simulink model "base_simulink"  (R2022a)
settings: Solver=FixedStepAuto  StartTime=0.0  StopTime=20  FixedStep=0.00005  MaxStep=1e-4  RelTol=1e-5
model workspace (MAT data in the model file):
  SL_ROS_VariableLengthArrays_MaxSizes : object (value not decoded)
undefined symbols (not defined in the file): position, position_SL_Info, sigbuilder_block, twist, X, Y, Z
libraries: sm_lib x128, nesl_utility x42, slpidlib x16, ros2lib x12, dspstat3 x2, dspsigops x1
(part 6 of 6)

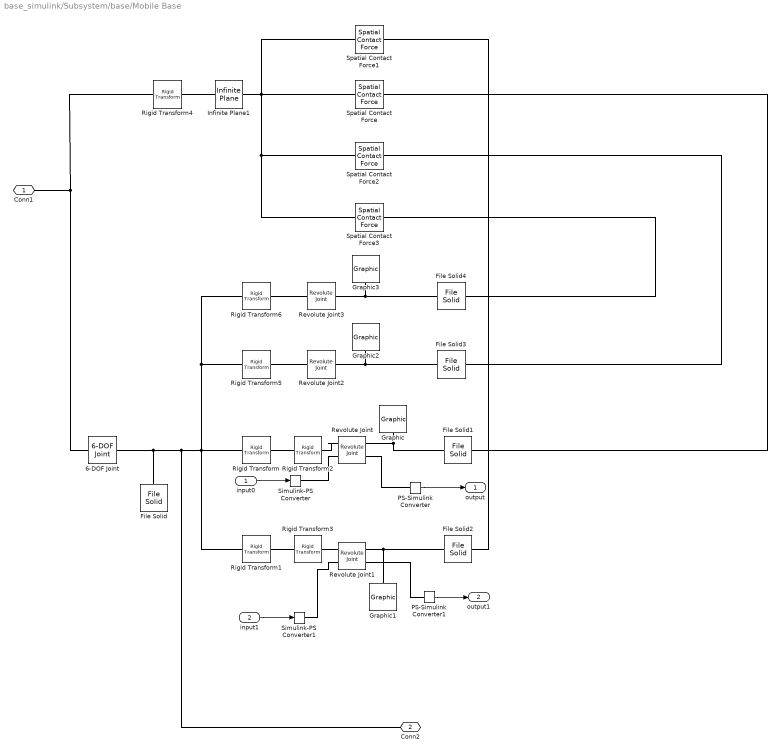
== system base_simulink/Subsystem/base/Mobile Base ==
  input0 : Inport
  input1 : Inport  Port=2
  6-DOF Joint : sm_lib/Joints/6-DOF Joint  JointMode=Normal  SenseConstraintForce=off  SenseConstraintForceX=off  SenseConstraintForceY=off  SenseConstraintForceZ=off  SenseConstraintTorque=off  SenseConstraintTorqueX=off  SenseConstraintTorqueY=off  SenseConstraintTorqueZ=off  SenseTotalForce=off  SenseTotalForceX=off  SenseTotalForceY=off  SenseTotalForceZ=off  SenseTotalTorque=off  SenseTotalTorqueX=off  SenseTotalTorqueY=off  SenseTotalTorqueZ=off  CompositeWrenchDir=FollowerOnBase  CompositeWrenchFrame=BaseFrame  PxEquilibriumPosition=0  PxEquilibriumPositionUnits=m  PxSpringStiffness=0  PxSpringStiffnessUnits=N/m  PxDampingCoefficient=0  PxDampingCoefficientUnits=N/(m/s)  PxTorqueActuationMode=NoTorque  PxMotionActuationMode=ComputedMotion  PxSensePosition=off  PxSenseVelocity=off  PxSenseAcceleration=off  PxSenseTorqueForce=off  PxSenseLowerLimitTorqueForce=off  PxSenseUpperLimitTorqueForce=off  PxLowerLimitSpecify=off  PxLowerLimitBound=-1  PxLowerLimitBoundUnits=m  PxLowerLimitStiffness=1e6  PxLowerLimitStiffnessUnits=N/m  PxLowerLimitDamping=1e3  PxLowerLimitDampingUnits=N/(m/s)  PxLowerLimitTransitionRegionWidth=1e-4  PxLowerLimitTransitionRegionWidthUnits=m  PxUpperLimitSpecify=off  PxUpperLimitBound=1  PxUpperLimitBoundUnits=m  PxUpperLimitStiffness=1e6  PxUpperLimitStiffnessUnits=N/m  PxUpperLimitDamping=1e3  PxUpperLimitDampingUnits=N/(m/s)  PxUpperLimitTransitionRegionWidth=1e-4  PxUpperLimitTransitionRegionWidthUnits=m  PxPositionTargetSpecify=off  PxPositionTargetPriority=High  PxPositionTargetValue=0  PxPositionTargetValueUnits=m  PxVelocityTargetSpecify=off  PxVelocityTargetPriority=High  PxVelocityTargetValue=0  PxVelocityTargetValueUnits=m/s  PyEquilibriumPosition=0  PyEquilibriumPositionUnits=m  PySpringStiffness=0  PySpringStiffnessUnits=N/m  PyDampingCoefficient=0  PyDampingCoefficientUnits=N/(m/s)  PyTorqueActuationMode=NoTorque  PyMotionActuationMode=ComputedMotion  PySensePosition=off  PySenseVelocity=off  PySenseAcceleration=off  PySenseTorqueForce=off  PySenseLowerLimitTorqueForce=off  PySenseUpperLimitTorqueForce=off  PyLowerLimitSpecify=off  PyLowerLimitBound=-1  PyLowerLimitBoundUnits=m  PyLowerLimitStiffness=1e6  PyLowerLimitStiffnessUnits=N/m  PyLowerLimitDamping=1e3  PyLowerLimitDampingUnits=N/(m/s)  PyLowerLimitTransitionRegionWidth=1e-4  PyLowerLimitTransitionRegionWidthUnits=m  PyUpperLimitSpecify=off  PyUpperLimitBound=1  PyUpperLimitBoundUnits=m  PyUpperLimitStiffness=1e6  PyUpperLimitStiffnessUnits=N/m  PyUpperLimitDamping=1e3  PyUpperLimitDampingUnits=N/(m/s)  PyUpperLimitTransitionRegionWidth=1e-4  PyUpperLimitTransitionRegionWidthUnits=m  PyPositionTargetSpecify=off  PyPositionTargetPriority=High  PyPositionTargetValue=0  PyPositionTargetValueUnits=m  PyVelocityTargetSpecify=off  PyVelocityTargetPriority=High  PyVelocityTargetValue=0  PyVelocityTargetValueUnits=m/s  PzEquilibriumPosition=0  PzEquilibriumPositionUnits=m  PzSpringStiffness=0  PzSpringStiffnessUnits=N/m  PzDampingCoefficient=0  PzDampingCoefficientUnits=N/(m/s)  PzTorqueActuationMode=NoTorque  PzMotionActuationMode=ComputedMotion  PzSensePosition=off  PzSenseVelocity=off  PzSenseAcceleration=off  PzSenseTorqueForce=off  PzSenseLowerLimitTorqueForce=off  PzSenseUpperLimitTorqueForce=off  PzLowerLimitSpecify=off  PzLowerLimitBound=-1  PzLowerLimitBoundUnits=m  PzLowerLimitStiffness=1e6  PzLowerLimitStiffnessUnits=N/m  PzLowerLimitDamping=1e3  PzLowerLimitDampingUnits=N/(m/s)  PzLowerLimitTransitionRegionWidth=1e-4  PzLowerLimitTransitionRegionWidthUnits=m  PzUpperLimitSpecify=off  PzUpperLimitBound=1  PzUpperLimitBoundUnits=m  PzUpperLimitStiffness=1e6  PzUpperLimitStiffnessUnits=N/m  PzUpperLimitDamping=1e3  PzUpperLimitDampingUnits=N/(m/s)  PzUpperLimitTransitionRegionWidth=1e-4  PzUpperLimitTransitionRegionWidthUnits=m  PzPositionTargetSpecify=off  PzPositionTargetPriority=High  PzPositionTargetValue=0  PzPositionTargetValueUnits=m  PzVelocityTargetSpecify=off  PzVelocityTargetPriority=High  PzVelocityTargetValue=0  PzVelocityTargetValueUnits=m/s  SphDefPosRotationMethod=None  SphDefPosRotationAngleUnits=deg  SphDefPosRotationStandardAxis=+Z  SphDefPosRotationAngle=0.0  SphDefPosRotationArbitraryAxis=[0 0 1]  SphDefPosFollAlignAxisA=+X  SphDefPosBaseAlignAxisA=+Y  SphDefPosFollAlignAxisB=+Y  SphDefPosBaseAlignAxisB=+Z  SphDefPosRotationSequenceAxes=FollowerAxes  SphDefPosRotationSequence=XYX  SphDefPosRotationSequenceAngles=[0 0 0]  SphDefPosRotationSequenceAnglesUnits=deg  SphDefPosRotationMatrix=[1 0 0; 0 1 0; 0 0 1]  SphEqPosRotationMethod=None  SphEqPosRotationAngleUnits=deg  SphEqPosRotationStandardAxis=+Z  SphEqPosRotationAngle=0.0  SphEqPosRotationArbitraryAxis=[0 0 1]  SphEqPosFollAlignAxisA=+X  SphEqPosBaseAlignAxisA=+Y  SphEqPosFollAlignAxisB=+Y  SphEqPosBaseAlignAxisB=+Z  SphEqPosRotationSequenceAxes=FollowerAxes  SphEqPosRotationSequence=XYX  SphEqPosRotationSequenceAngles=[0 0 0]  SphEqPosRotationSequenceAnglesUnits=deg  SphEqPosRotationMatrix=[1 0 0; 0 1 0; 0 0 1]  SphSpringStiffness=0  SphSpringStiffnessUnits=N*m/deg  SphDampingCoefficient=0  SphDampingCoefficientUnits=N*m/(deg/s)  SphActuateTorqueX=off  SphActuateTorqueY=off  SphActuateTorqueZ=off  SphActuateTorque=off  SphTorqueActuationMode=NoTorque  SphMotionActuationMode=ComputedMotion  SphActuationFrame=BaseFrame  SphSensePosition=off  SphSenseVelocityX=off  SphSenseVelocityY=off  SphSenseVelocityZ=off  SphSenseVelocity=off  SphSenseAccelerationX=off  SphSenseAccelerationY=off  SphSenseAccelerationZ=off  SphSenseAcceleration=off  SphSenseTorqueX=off  SphSenseTorqueY=off  SphSenseTorqueZ=off  SphSenseTorqueForce=off  SphSenseLowerLimitTorqueMag=off  SphSenseUpperLimitTorqueMag=off  SphSensingFrame=BaseFrame  SphLowerLimitSpecify=off  SphLowerLimitBound=15  SphLowerLimitBoundUnits=deg  SphLowerLimitStiffness=1e4  SphLowerLimitStiffnessUnits=N*m/deg  SphLowerLimitDamping=10  SphLowerLimitDampingUnits=N*m/(deg/s)  SphLowerLimitTransitionRegionWidth=0.1  SphLowerLimitTransitionRegionWidthUnits=deg  SphUpperLimitSpecify=off  SphUpperLimitBound=45  SphUpperLimitBoundUnits=deg  SphUpperLimitStiffness=1e4  SphUpperLimitStiffnessUnits=N*m/deg  SphUpperLimitDamping=10  SphUpperLimitDampingUnits=N*m/(deg/s)  SphUpperLimitTransitionRegionWidth=0.1  SphUpperLimitTransitionRegionWidthUnits=deg  SphPositionTargetRotationMethod=None  SphPositionTargetRotationAngleUnits=deg  SphPositionTargetRotationStandardAxis=+Z  SphPositionTargetRotationAngle=0.0  SphPositionTargetRotationArbitraryAxis=[0 0 1]  SphPositionTargetFollAlignAxisA=+X  SphPositionTargetBaseAlignAxisA=+Y  SphPositionTargetFollAlignAxisB=+Y  SphPositionTargetBaseAlignAxisB=+Z  SphPositionTargetRotationSequenceAxes=FollowerAxes  SphPositionTargetRotationSequence=XYX  SphPositionTargetRotationSequenceAngles=[0 0 0]  SphPositionTargetRotationSequenceAnglesUnits=deg  SphPositionTargetRotationMatrix=[1 0 0; 0 1 0; 0 0 1]  SphPositionTargetSpecify=off  SphPositionTargetPriority=High  SphVelocityTargetValue=[0 0 0]  SphVelocityTargetValueUnits=deg/s  SphVelocityTargetSpecify=off  SphVelocityTargetPriority=High  SphVelocityTargetInFollowerFrame=on
  File Solid : sm_lib/Body Elements/File Solid  ExtGeomFileName=C:\Users\matas\Desktop\FIBO4\FRA502MBSE\BASE_simulink\BASE_simulink\chassis.step  UnitType=FromFile  ExtGeomFileUnits=m  StepReaderType=HEX  ExportConvexHullGeometry=off  InertiaType=Custom  Mass=45.683  MassUnits=kg  CenterOfMass=[-117.99 2.46 415.85]  CenterOfMassUnits=mm  MomentsOfInertia=[16.23572765580 17.36819929236 2.01273191058]  MomentsOfInertiaUnits=kg*m^2  ProductsOfInertia=[0.10365361699 1.80624053893 0.02552226667]  ProductsOfInertiaUnits=kg*m^2  BasedOnType=DensityFromFile  Density=1000  DensityUnits=kg/m^3  DoExposeReferenceFrame=on  SerializedFrames=<Frames/>  GraphicType=FromGeometry  MarkerShape=Sphere  MarkerSize=10  GraphicVisPropType=SimpleVisualProperties  GraphicDiffuseColor=[0.5 0.5 0.5]  GraphicSpecularColor=[0.5 0.5 0.5 1.0]  GraphicAmbientColor=[0.15 0.15 0.15 1.0]  GraphicEmissiveColor=[0.0 0.0 0.0 1.0]  GraphicShininess=75  GraphicOpacity=1.0
  File Solid1 : sm_lib/Body Elements/File Solid  ExtGeomFileName=C:\Users\matas\Desktop\FIBO4\FRA502MBSE\BASE_simulink\BASE_simulink\wheel.step  UnitType=FromFile  ExtGeomFileUnits=m  StepReaderType=HEX  ExportConvexHullGeometry=on  InertiaType=CalculateFromGeometry  Mass=0.5  MassUnits=kg  CenterOfMass=[0 0 0]  CenterOfMassUnits=m  MomentsOfInertia=[1 1 1]  MomentsOfInertiaUnits=kg*m^2  ProductsOfInertia=[0 0 0]  ProductsOfInertiaUnits=kg*m^2  BasedOnType=Mass  Density=1000  DensityUnits=kg/m^3  DoExposeReferenceFrame=on  SerializedFrames=<Frames/>  GraphicType=FromGeometry  MarkerShape=Sphere  MarkerSize=10  GraphicVisPropType=SimpleVisualProperties  GraphicDiffuseColor=[0.5 0.5 0.5]  GraphicSpecularColor=[0.5 0.5 0.5 1.0]  GraphicAmbientColor=[0.15 0.15 0.15 1.0]  GraphicEmissiveColor=[0.0 0.0 0.0 1.0]  GraphicShininess=75  GraphicOpacity=1.0
  File Solid2 : sm_lib/Body Elements/File Solid  ExtGeomFileName=C:\Users\matas\Desktop\FIBO4\FRA502MBSE\BASE_simulink\BASE_simulink\wheel.step  UnitType=FromFile  ExtGeomFileUnits=m  StepReaderType=HEX  ExportConvexHullGeometry=on  InertiaType=CalculateFromGeometry  Mass=0.5  MassUnits=kg  CenterOfMass=[0 0 0]  CenterOfMassUnits=m  MomentsOfInertia=[1 1 1]  MomentsOfInertiaUnits=kg*m^2  ProductsOfInertia=[0 0 0]  ProductsOfInertiaUnits=kg*m^2  BasedOnType=Mass  Density=1000  DensityUnits=kg/m^3  DoExposeReferenceFrame=on  SerializedFrames=<Frames/>  GraphicType=FromGeometry  MarkerShape=Sphere  MarkerSize=10  GraphicVisPropType=SimpleVisualProperties  GraphicDiffuseColor=[0.5 0.5 0.5]  GraphicSpecularColor=[0.5 0.5 0.5 1.0]  GraphicAmbientColor=[0.15 0.15 0.15 1.0]  GraphicEmissiveColor=[0.0 0.0 0.0 1.0]  GraphicShininess=75  GraphicOpacity=1.0
  File Solid3 : sm_lib/Body Elements/File Solid  ExtGeomFileName=C:\Users\matas\Desktop\FIBO4\FRA502MBSE\BASE_simulink\BASE_simulink\caster wheel.step  UnitType=FromFile  ExtGeomFileUnits=m  StepReaderType=HEX  ExportConvexHullGeometry=on  InertiaType=CalculateFromGeometry  Mass=1  MassUnits=kg  CenterOfMass=[0 0 0]  CenterOfMassUnits=m  MomentsOfInertia=[1 1 1]  MomentsOfInertiaUnits=kg*m^2  ProductsOfInertia=[0 0 0]  ProductsOfInertiaUnits=kg*m^2  BasedOnType=Mass  Density=1000  DensityUnits=kg/m^3  DoExposeReferenceFrame=on  SerializedFrames=<Frames/>  GraphicType=FromGeometry  MarkerShape=Sphere  MarkerSize=10  GraphicVisPropType=SimpleVisualProperties  GraphicDiffuseColor=[0.5 0.5 0.5]  GraphicSpecularColor=[0.5 0.5 0.5 1.0]  GraphicAmbientColor=[0.15 0.15 0.15 1.0]  GraphicEmissiveColor=[0.0 0.0 0.0 1.0]  GraphicShininess=75  GraphicOpacity=1.0
  File Solid4 : sm_lib/Body Elements/File Solid  ExtGeomFileName=C:\Users\matas\Desktop\FIBO4\FRA502MBSE\BASE_simulink\BASE_simulink\caster wheel.step  UnitType=FromFile  ExtGeomFileUnits=m  StepReaderType=HEX  ExportConvexHullGeometry=on  InertiaType=CalculateFromGeometry  Mass=1  MassUnits=kg  CenterOfMass=[0 0 0]  CenterOfMassUnits=m  MomentsOfInertia=[1 1 1]  MomentsOfInertiaUnits=kg*m^2  ProductsOfInertia=[0 0 0]  ProductsOfInertiaUnits=kg*m^2  BasedOnType=Mass  Density=1000  DensityUnits=kg/m^3  DoExposeReferenceFrame=on  SerializedFrames=<Frames/>  GraphicType=FromGeometry  MarkerShape=Sphere  MarkerSize=10  GraphicVisPropType=SimpleVisualProperties  GraphicDiffuseColor=[0.5 0.5 0.5]  GraphicSpecularColor=[0.5 0.5 0.5 1.0]  GraphicAmbientColor=[0.15 0.15 0.15 1.0]  GraphicEmissiveColor=[0.0 0.0 0.0 1.0]  GraphicShininess=75  GraphicOpacity=1.0
  Graphic : sm_lib/Body Elements/Graphic  GraphicType=Marker  MarkerShape=Frame  MarkerSize=20  GraphicVisPropType=SimpleVisualProperties  GraphicDiffuseColor=[0 1 0]  GraphicSpecularColor=[0.5 0.5 0.5 1.0]  GraphicAmbientColor=[0.15 0.15 0.15 1.0]  GraphicEmissiveColor=[0.0 0.0 0.0 1.0]  GraphicShininess=75  GraphicOpacity=1.0
  Graphic1 : sm_lib/Body Elements/Graphic  GraphicType=Marker  MarkerShape=Frame  MarkerSize=20  GraphicVisPropType=SimpleVisualProperties  GraphicDiffuseColor=[1 0 0]  GraphicSpecularColor=[0.5 0.5 0.5 1.0]  GraphicAmbientColor=[0.15 0.15 0.15 1.0]  GraphicEmissiveColor=[0.0 0.0 0.0 1.0]  GraphicShininess=75  GraphicOpacity=1.0
  Graphic2 : sm_lib/Body Elements/Graphic  GraphicType=Marker  MarkerShape=Frame  MarkerSize=20  GraphicVisPropType=SimpleVisualProperties  GraphicDiffuseColor=[1 0 0]  GraphicSpecularColor=[0.5 0.5 0.5 1.0]  GraphicAmbientColor=[0.15 0.15 0.15 1.0]  GraphicEmissiveColor=[0.0 0.0 0.0 1.0]  GraphicShininess=75  GraphicOpacity=1.0
  Graphic3 : sm_lib/Body Elements/Graphic  GraphicType=Marker  MarkerShape=Frame  MarkerSize=20  GraphicVisPropType=SimpleVisualProperties  GraphicDiffuseColor=[1 0 0]  GraphicSpecularColor=[0.5 0.5 0.5 1.0]  GraphicAmbientColor=[0.15 0.15 0.15 1.0]  GraphicEmissiveColor=[0.0 0.0 0.0 1.0]  GraphicShininess=75  GraphicOpacity=1.0
  Infinite Plane1 : sm_lib/Curves and Surfaces/Infinite Plane  GraphicType=Rectangle  GraphicPlaneWidth=10  GraphicPlaneWidthUnits=m  GraphicPlaneHeight=10  GraphicPlaneHeightUnits=m  GraphicVisPropType=SimpleVisualProperties  GraphicDiffuseColor=[0.149 0.149 0.149]  GraphicOpacity=0.25  GraphicSpecularColor=[0.5 0.5 0.5 1.0]  GraphicAmbientColor=[0.15 0.15 0.15 1.0]  GraphicEmissiveColor=[0.0 0.0 0.0 1.0]  GraphicShininess=75
  PS-Simulink Converter : nesl_utility/PS-Simulink Converter  PhysicalDomain=network_engine_domain  SubClassName=ps_output  LeftPortType=input  RightPortType=output  PseudoPeriodic=off  Frequencies=[]  Unit=inherit  AffineConversion=off
      settings: SourceProductBaseCode=SS,PW,VE
  PS-Simulink Converter1 : nesl_utility/PS-Simulink Converter  PhysicalDomain=network_engine_domain  SubClassName=ps_output  LeftPortType=input  RightPortType=output  PseudoPeriodic=off  Frequencies=[]  Unit=inherit  AffineConversion=off
      settings: SourceProductBaseCode=SS,PW,VE
  Revolute Joint : sm_lib/Joints/Revolute Joint  JointMode=Normal  SenseConstraintForce=off  SenseConstraintForceX=off  SenseConstraintForceY=off  SenseConstraintForceZ=off  SenseConstraintTorque=off  SenseConstraintTorqueX=off  SenseConstraintTorqueY=off  SenseConstraintTorqueZ=off  SenseTotalForce=off  SenseTotalForceX=off  SenseTotalForceY=off  SenseTotalForceZ=off  SenseTotalTorque=off  SenseTotalTorqueX=off  SenseTotalTorqueY=off  SenseTotalTorqueZ=off  CompositeWrenchDir=FollowerOnBase  CompositeWrenchFrame=BaseFrame  EquilibriumPosition=0  EquilibriumPositionUnits=deg  SpringStiffness=0  SpringStiffnessUnits=N*m/deg  DampingCoefficient=0  DampingCoefficientUnits=N*m/(deg/s)  TorqueActuationMode=InputTorque  MotionActuationMode=ComputedMotion  SensePosition=on  SenseVelocity=off  SenseAcceleration=off  SenseTorqueForce=off  SenseLowerLimitTorqueForce=off  SenseUpperLimitTorqueForce=off  LowerLimitSpecify=off  LowerLimitBound=-90  LowerLimitBoundUnits=deg  LowerLimitStiffness=1e4  LowerLimitStiffnessUnits=N*m/deg  LowerLimitDamping=10  LowerLimitDampingUnits=N*m/(deg/s)  LowerLimitTransitionRegionWidth=0.1  LowerLimitTransitionRegionWidthUnits=deg  UpperLimitSpecify=off  UpperLimitBound=90  UpperLimitBoundUnits=deg  UpperLimitStiffness=1e4  UpperLimitStiffnessUnits=N*m/deg  UpperLimitDamping=10  UpperLimitDampingUnits=N*m/(deg/s)  UpperLimitTransitionRegionWidth=0.1  UpperLimitTransitionRegionWidthUnits=deg  PositionTargetSpecify=off  PositionTargetPriority=High  PositionTargetValue=0  PositionTargetValueUnits=deg  VelocityTargetSpecify=off  VelocityTargetPriority=High  VelocityTargetValue=0  VelocityTargetValueUnits=deg/s
  Revolute Joint1 : sm_lib/Joints/Revolute Joint  JointMode=Normal  SenseConstraintForce=off  SenseConstraintForceX=off  SenseConstraintForceY=off  SenseConstraintForceZ=off  SenseConstraintTorque=off  SenseConstraintTorqueX=off  SenseConstraintTorqueY=off  SenseConstraintTorqueZ=off  SenseTotalForce=off  SenseTotalForceX=off  SenseTotalForceY=off  SenseTotalForceZ=off  SenseTotalTorque=off  SenseTotalTorqueX=off  SenseTotalTorqueY=off  SenseTotalTorqueZ=off  CompositeWrenchDir=FollowerOnBase  CompositeWrenchFrame=BaseFrame  EquilibriumPosition=0  EquilibriumPositionUnits=deg  SpringStiffness=0  SpringStiffnessUnits=N*m/deg  DampingCoefficient=0  DampingCoefficientUnits=N*m/(deg/s)  TorqueActuationMode=InputTorque  MotionActuationMode=ComputedMotion  SensePosition=on  SenseVelocity=off  SenseAcceleration=off  SenseTorqueForce=off  SenseLowerLimitTorqueForce=off  SenseUpperLimitTorqueForce=off  LowerLimitSpecify=off  LowerLimitBound=-90  LowerLimitBoundUnits=deg  LowerLimitStiffness=1e4  LowerLimitStiffnessUnits=N*m/deg  LowerLimitDamping=10  LowerLimitDampingUnits=N*m/(deg/s)  LowerLimitTransitionRegionWidth=0.1  LowerLimitTransitionRegionWidthUnits=deg  UpperLimitSpecify=off  UpperLimitBound=90  UpperLimitBoundUnits=deg  UpperLimitStiffness=1e4  UpperLimitStiffnessUnits=N*m/deg  UpperLimitDamping=10  UpperLimitDampingUnits=N*m/(deg/s)  UpperLimitTransitionRegionWidth=0.1  UpperLimitTransitionRegionWidthUnits=deg  PositionTargetSpecify=off  PositionTargetPriority=High  PositionTargetValue=0  PositionTargetValueUnits=deg  VelocityTargetSpecify=off  VelocityTargetPriority=High  VelocityTargetValue=0  VelocityTargetValueUnits=deg/s
  Revolute Joint2 : sm_lib/Joints/Revolute Joint  JointMode=Normal  SenseConstraintForce=off  SenseConstraintForceX=off  SenseConstraintForceY=off  SenseConstraintForceZ=off  SenseConstraintTorque=off  SenseConstraintTorqueX=off  SenseConstraintTorqueY=off  SenseConstraintTorqueZ=off  SenseTotalForce=off  SenseTotalForceX=off  SenseTotalForceY=off  SenseTotalForceZ=off  SenseTotalTorque=off  SenseTotalTorqueX=off  SenseTotalTorqueY=off  SenseTotalTorqueZ=off  CompositeWrenchDir=FollowerOnBase  CompositeWrenchFrame=BaseFrame  EquilibriumPosition=0  EquilibriumPositionUnits=deg  SpringStiffness=0  SpringStiffnessUnits=N*m/deg  DampingCoefficient=0  DampingCoefficientUnits=N*m/(deg/s)  TorqueActuationMode=NoTorque  MotionActuationMode=ComputedMotion  SensePosition=off  SenseVelocity=off  SenseAcceleration=off  SenseTorqueForce=off  SenseLowerLimitTorqueForce=off  SenseUpperLimitTorqueForce=off  LowerLimitSpecify=off  LowerLimitBound=-90  LowerLimitBoundUnits=deg  LowerLimitStiffness=1e4  LowerLimitStiffnessUnits=N*m/deg  LowerLimitDamping=10  LowerLimitDampingUnits=N*m/(deg/s)  LowerLimitTransitionRegionWidth=0.1  LowerLimitTransitionRegionWidthUnits=deg  UpperLimitSpecify=off  UpperLimitBound=90  UpperLimitBoundUnits=deg  UpperLimitStiffness=1e4  UpperLimitStiffnessUnits=N*m/deg  UpperLimitDamping=10  UpperLimitDampingUnits=N*m/(deg/s)  UpperLimitTransitionRegionWidth=0.1  UpperLimitTransitionRegionWidthUnits=deg  PositionTargetSpecify=off  PositionTargetPriority=High  PositionTargetValue=0  PositionTargetValueUnits=deg  VelocityTargetSpecify=off  VelocityTargetPriority=High  VelocityTargetValue=0  VelocityTargetValueUnits=deg/s
  Revolute Joint3 : sm_lib/Joints/Revolute Joint  JointMode=Normal  SenseConstraintForce=off  SenseConstraintForceX=off  SenseConstraintForceY=off  SenseConstraintForceZ=off  SenseConstraintTorque=off  SenseConstraintTorqueX=off  SenseConstraintTorqueY=off  SenseConstraintTorqueZ=off  SenseTotalForce=off  SenseTotalForceX=off  SenseTotalForceY=off  SenseTotalForceZ=off  SenseTotalTorque=off  SenseTotalTorqueX=off  SenseTotalTorqueY=off  SenseTotalTorqueZ=off  CompositeWrenchDir=FollowerOnBase  CompositeWrenchFrame=BaseFrame  EquilibriumPosition=0  EquilibriumPositionUnits=deg  SpringStiffness=0  SpringStiffnessUnits=N*m/deg  DampingCoefficient=0  DampingCoefficientUnits=N*m/(deg/s)  TorqueActuationMode=NoTorque  MotionActuationMode=ComputedMotion  SensePosition=off  SenseVelocity=off  SenseAcceleration=off  SenseTorqueForce=off  SenseLowerLimitTorqueForce=off  SenseUpperLimitTorqueForce=off  LowerLimitSpecify=off  LowerLimitBound=-90  LowerLimitBoundUnits=deg  LowerLimitStiffness=1e4  LowerLimitStiffnessUnits=N*m/deg  LowerLimitDamping=10  LowerLimitDampingUnits=N*m/(deg/s)  LowerLimitTransitionRegionWidth=0.1  LowerLimitTransitionRegionWidthUnits=deg  UpperLimitSpecify=off  UpperLimitBound=90  UpperLimitBoundUnits=deg  UpperLimitStiffness=1e4  UpperLimitStiffnessUnits=N*m/deg  UpperLimitDamping=10  UpperLimitDampingUnits=N*m/(deg/s)  UpperLimitTransitionRegionWidth=0.1  UpperLimitTransitionRegionWidthUnits=deg  PositionTargetSpecify=off  PositionTargetPriority=High  PositionTargetValue=0  PositionTargetValueUnits=deg  VelocityTargetSpecify=off  VelocityTargetPriority=High  VelocityTargetValue=0  VelocityTargetValueUnits=deg/s
  Rigid Transform : sm_lib/Frames and Transforms/Rigid Transform  TranslationMethod=Cartesian  TranslationStandardOffset=0  TranslationLengthUnit=mm  TranslationStandardAxis=+Z  TranslationCartesianOffset=[0 125 0]  TranslationROffset=0  TranslationROffsetUnits=m  TranslationZOffset=0  TranslationZOffsetUnits=m  TranslationThetaOffset=0  TranslationThetaOffsetUnits=deg  RotationMethod=None  RotationAngleUnits=deg  RotationStandardAxis=+Z  RotationAngle=0.0  RotationArbitraryAxis=[0 0 1]  FollAlignAxisA=+X  BaseAlignAxisA=+Y  FollAlignAxisB=+Y  BaseAlignAxisB=+Z  RotationSequenceAxes=FollowerAxes  RotationSequence=XYX  RotationSequenceAngles=[0 0 0]  RotationSequenceAnglesUnits=deg  RotationMatrix=[1 0 0; 0 1 0; 0 0 1]
  Rigid Transform1 : sm_lib/Frames and Transforms/Rigid Transform  TranslationMethod=Cartesian  TranslationStandardOffset=0  TranslationLengthUnit=mm  TranslationStandardAxis=+Z  TranslationCartesianOffset=[0 -125 0]  TranslationROffset=0  TranslationROffsetUnits=m  TranslationZOffset=0  TranslationZOffsetUnits=m  TranslationThetaOffset=0  TranslationThetaOffsetUnits=deg  RotationMethod=None  RotationAngleUnits=deg  RotationStandardAxis=+Z  RotationAngle=0.0  RotationArbitraryAxis=[0 0 1]  FollAlignAxisA=+X  BaseAlignAxisA=+Y  FollAlignAxisB=+Y  BaseAlignAxisB=+Z  RotationSequenceAxes=FollowerAxes  RotationSequence=XYX  RotationSequenceAngles=[0 0 0]  RotationSequenceAnglesUnits=deg  RotationMatrix=[1 0 0; 0 1 0; 0 0 1]
  Rigid Transform2 : sm_lib/Frames and Transforms/Rigid Transform  TranslationMethod=None  TranslationStandardOffset=0  TranslationLengthUnit=mm  TranslationStandardAxis=+Z  TranslationCartesianOffset=[0 125 0]  TranslationROffset=0  TranslationROffsetUnits=m  TranslationZOffset=0  TranslationZOffsetUnits=m  TranslationThetaOffset=0  TranslationThetaOffsetUnits=deg  RotationMethod=StandardAxis  RotationAngleUnits=deg  RotationStandardAxis=-X  RotationAngle=90  RotationArbitraryAxis=[0 0 1]  FollAlignAxisA=+X  BaseAlignAxisA=+Y  FollAlignAxisB=+Y  BaseAlignAxisB=+Z  RotationSequenceAxes=FollowerAxes  RotationSequence=XYX  RotationSequenceAngles=[0 0 0]  RotationSequenceAnglesUnits=deg  RotationMatrix=[1 0 0; 0 1 0; 0 0 1]
  Rigid Transform3 : sm_lib/Frames and Transforms/Rigid Transform  TranslationMethod=None  TranslationStandardOffset=0  TranslationLengthUnit=mm  TranslationStandardAxis=+Z  TranslationCartesianOffset=[0 125 0]  TranslationROffset=0  TranslationROffsetUnits=m  TranslationZOffset=0  TranslationZOffsetUnits=m  TranslationThetaOffset=0  TranslationThetaOffsetUnits=deg  RotationMethod=StandardAxis  RotationAngleUnits=deg  RotationStandardAxis=-X  RotationAngle=90  RotationArbitraryAxis=[0 0 1]  FollAlignAxisA=+X  BaseAlignAxisA=+Y  FollAlignAxisB=+Y  BaseAlignAxisB=+Z  RotationSequenceAxes=FollowerAxes  RotationSequence=XYX  RotationSequenceAngles=[0 0 0]  RotationSequenceAnglesUnits=deg  RotationMatrix=[1 0 0; 0 1 0; 0 0 1]
  Rigid Transform4 : sm_lib/Frames and Transforms/Rigid Transform  TranslationMethod=Cartesian  TranslationStandardOffset=0  TranslationLengthUnit=mm  TranslationStandardAxis=+Z  TranslationCartesianOffset=[0 0 -100]  TranslationROffset=0  TranslationROffsetUnits=m  TranslationZOffset=0  TranslationZOffsetUnits=m  TranslationThetaOffset=0  TranslationThetaOffsetUnits=deg  RotationMethod=None  RotationAngleUnits=deg  RotationStandardAxis=+Z  RotationAngle=0.0  RotationArbitraryAxis=[0 0 1]  FollAlignAxisA=+X  BaseAlignAxisA=+Y  FollAlignAxisB=+Y  BaseAlignAxisB=+Z  RotationSequenceAxes=FollowerAxes  RotationSequence=XYX  RotationSequenceAngles=[0 0 0]  RotationSequenceAnglesUnits=deg  RotationMatrix=[1 0 0; 0 1 0; 0 0 1]
  Rigid Transform5 : sm_lib/Frames and Transforms/Rigid Transform  TranslationMethod=Cartesian  TranslationStandardOffset=0  TranslationLengthUnit=mm  TranslationStandardAxis=+Z  TranslationCartesianOffset=[-245 -175 55]  TranslationROffset=0  TranslationROffsetUnits=m  TranslationZOffset=0  TranslationZOffsetUnits=m  TranslationThetaOffset=0  TranslationThetaOffsetUnits=deg  RotationMethod=None  RotationAngleUnits=deg  RotationStandardAxis=+Z  RotationAngle=0.0  RotationArbitraryAxis=[0 0 1]  FollAlignAxisA=+X  BaseAlignAxisA=+Y  FollAlignAxisB=+Y  BaseAlignAxisB=+Z  RotationSequenceAxes=FollowerAxes  RotationSequence=XYX  RotationSequenceAngles=[0 0 0]  RotationSequenceAnglesUnits=deg  RotationMatrix=[1 0 0; 0 1 0; 0 0 1]
  Rigid Transform6 : sm_lib/Frames and Transforms/Rigid Transform  TranslationMethod=Cartesian  TranslationStandardOffset=0  TranslationLengthUnit=mm  TranslationStandardAxis=+Z  TranslationCartesianOffset=[-245 175 55]  TranslationROffset=0  TranslationROffsetUnits=m  TranslationZOffset=0  TranslationZOffsetUnits=m  TranslationThetaOffset=0  TranslationThetaOffsetUnits=deg  RotationMethod=None  RotationAngleUnits=deg  RotationStandardAxis=+Z  RotationAngle=0.0  RotationArbitraryAxis=[0 0 1]  FollAlignAxisA=+X  BaseAlignAxisA=+Y  FollAlignAxisB=+Y  BaseAlignAxisB=+Z  RotationSequenceAxes=FollowerAxes  RotationSequence=XYX  RotationSequenceAngles=[0 0 0]  RotationSequenceAnglesUnits=deg  RotationMatrix=[1 0 0; 0 1 0; 0 0 1]
  Simulink-PS Converter : nesl_utility/Simulink-PS Converter  PhysicalDomain=network_engine_domain  SubClassName=ps_input  LeftPortType=input  RightPortType=output  PseudoPeriodic=off  Frequencies=[]  NoiseDistribution=none  NoiseParameters=[]  Unit=1  AffineConversion=off  FilteringAndDerivatives=filter  SimscapeFilterOrder=2  InputFilterTimeConstant=0.001  UdotUserProvided=0
      settings: SourceProductBaseCode=SS,PW,VE
  Simulink-PS Converter1 : nesl_utility/Simulink-PS Converter  PhysicalDomain=network_engine_domain  SubClassName=ps_input  LeftPortType=input  RightPortType=output  PseudoPeriodic=off  Frequencies=[]  NoiseDistribution=none  NoiseParameters=[]  Unit=1  AffineConversion=off  FilteringAndDerivatives=filter  SimscapeFilterOrder=2  InputFilterTimeConstant=0.001  UdotUserProvided=0
      settings: SourceProductBaseCode=SS,PW,VE
  Spatial Contact Force : sm_lib/Forces and Torques/Spatial Contact Force  CoefficientOfDynamicFriction=0.3  CoefficientOfStaticFriction=0.5  SenseContactBaseRotation=off  SenseContactBaseTranslation=off  NormalDamping=1e3  NormalDampingUnits=N/(m/s)  SenseContactFollowerRotation=off  SenseContactFollowerTranslation=off  SenseContactSignal=off  NormalStiffness=1e6  NormalStiffnessUnits=N/m  FrictionalCriticalVelocity=1e-3  FrictionalCriticalVelocityUnits=m/s  ZeroCrossDetectContactStartAndEnd=off  FrictionType=SmoothStickSlip  SenseFrictionalForceMagnitude=off  SenseNormalForceMagnitude=off  NormalForceType=SmoothSpringDamper  SenseNormalVelocity=off  SenseSeparationDistance=off  SenseTangentialVelocity=off  SenseTangentialVelocityMagnitude=off  NormalTransitionRegionWidth=1e-4  NormalTransitionRegionWidthUnits=m
  Spatial Contact Force1 : sm_lib/Forces and Torques/Spatial Contact Force  CoefficientOfDynamicFriction=0.3  CoefficientOfStaticFriction=0.5  SenseContactBaseRotation=off  SenseContactBaseTranslation=off  NormalDamping=1e3  NormalDampingUnits=N/(m/s)  SenseContactFollowerRotation=off  SenseContactFollowerTranslation=off  SenseContactSignal=off  NormalStiffness=1e6  NormalStiffnessUnits=N/m  FrictionalCriticalVelocity=1e-3  FrictionalCriticalVelocityUnits=m/s  ZeroCrossDetectContactStartAndEnd=off  FrictionType=SmoothStickSlip  SenseFrictionalForceMagnitude=off  SenseNormalForceMagnitude=off  NormalForceType=SmoothSpringDamper  SenseNormalVelocity=off  SenseSeparationDistance=off  SenseTangentialVelocity=off  SenseTangentialVelocityMagnitude=off  NormalTransitionRegionWidth=1e-4  NormalTransitionRegionWidthUnits=m
  Spatial Contact Force2 : sm_lib/Forces and Torques/Spatial Contact Force  CoefficientOfDynamicFriction=0  CoefficientOfStaticFriction=0  SenseContactBaseRotation=off  SenseContactBaseTranslation=off  NormalDamping=1e3  NormalDampingUnits=N/(m/s)  SenseContactFollowerRotation=off  SenseContactFollowerTranslation=off  SenseContactSignal=off  NormalStiffness=1e6  NormalStiffnessUnits=N/m  FrictionalCriticalVelocity=1e-3  FrictionalCriticalVelocityUnits=m/s  ZeroCrossDetectContactStartAndEnd=off  FrictionType=SmoothStickSlip  SenseFrictionalForceMagnitude=off  SenseNormalForceMagnitude=off  NormalForceType=SmoothSpringDamper  SenseNormalVelocity=off  SenseSeparationDistance=off  SenseTangentialVelocity=off  SenseTangentialVelocityMagnitude=off  NormalTransitionRegionWidth=1e-4  NormalTransitionRegionWidthUnits=m
  Spatial Contact Force3 : sm_lib/Forces and Torques/Spatial Contact Force  CoefficientOfDynamicFriction=0  CoefficientOfStaticFriction=0  SenseContactBaseRotation=off  SenseContactBaseTranslation=off  NormalDamping=1e3  NormalDampingUnits=N/(m/s)  SenseContactFollowerRotation=off  SenseContactFollowerTranslation=off  SenseContactSignal=off  NormalStiffness=1e6  NormalStiffnessUnits=N/m  FrictionalCriticalVelocity=1e-3  FrictionalCriticalVelocityUnits=m/s  ZeroCrossDetectContactStartAndEnd=off  FrictionType=SmoothStickSlip  SenseFrictionalForceMagnitude=off  SenseNormalForceMagnitude=off  NormalForceType=SmoothSpringDamper  SenseNormalVelocity=off  SenseSeparationDistance=off  SenseTangentialVelocity=off  SenseTangentialVelocityMagnitude=off  NormalTransitionRegionWidth=1e-4  NormalTransitionRegionWidthUnits=m
  Conn1 : PMIOPort  Side=Left
  Conn2 : PMIOPort  Port=2  Side=Right
  output : Outport
  output1 : Outport  Port=2
  wires:
  PS-Simulink Converter1/1 -> output1/1
  PS-Simulink Converter/1 -> output/1
  input0/1 -> Simulink-PS Converter/1
  input1/1 -> Simulink-PS Converter1/1
  connections:
  Spatial Contact Force1/RConn1 -- File Solid2/LConn1
  Graphic/RConn1 -- File Solid1/RConn1 -- Revolute Joint/RConn1
  Graphic2/RConn1 -- File Solid3/RConn1 -- Revolute Joint2/RConn1
  Revolute Joint3/RConn1 -- Graphic3/RConn1 -- File Solid4/RConn1
  Rigid Transform2/LConn1 -- Rigid Transform/RConn1
  Spatial Contact Force/LConn1 -- Infinite Plane1/RConn1 -- Spatial Contact Force3/LConn1 -- Spatial Contact Force2/LConn1 -- Spatial Contact Force1/LConn1
  Rigid Transform4/LConn1 -- Conn1/RConn1 -- 6-DOF Joint/LConn1
  Rigid Transform6/LConn1 -- Rigid Transform5/LConn1 -- Conn2/RConn1 -- File Solid/RConn1 -- 6-DOF Joint/RConn1 -- Rigid Transform/LConn1 -- Rigid Transform1/LConn1
  Infinite Plane1/LConn1 -- Rigid Transform4/RConn1
  Revolute Joint/LConn2 -- Simulink-PS Converter/RConn1
  Graphic1/RConn1 -- File Solid2/RConn1 -- Revolute Joint1/RConn1
  Spatial Contact Force3/RConn1 -- File Solid4/LConn1
  File Solid1/LConn1 -- Spatial Contact Force/RConn1
  Revolute Joint1/LConn1 -- Rigid Transform3/RConn1
  Revolute Joint/LConn1 -- Rigid Transform2/RConn1
  Revolute Joint/RConn2 -- PS-Simulink Converter/LConn1
  Simulink-PS Converter1/RConn1 -- Revolute Joint1/LConn2
  File Solid3/LConn1 -- Spatial Contact Force2/RConn1
  Revolute Joint2/LConn1 -- Rigid Transform5/RConn1
  Rigid Transform3/LConn1 -- Rigid Transform1/RConn1
  Revolute Joint3/LConn1 -- Rigid Transform6/RConn1
  Revolute Joint1/RConn2 -- PS-Simulink Converter1/LConn1

== system base_simulink/HouseM8/base/Manipulator/External Load ==
  Brick Solid : sm_lib/Body Elements/Brick Solid  GraphicAmbientColor=[0.15 0.15 0.15 1.0]  BasedOnType=Mass  BrickDimensions=[50 50 50]  BrickDimensionUnits=mm  CenterOfMass=[0 0 0]  CenterOfMassUnits=m  GraphicDiffuseColor=[0.5 0.5 0.5]  Density=1000  DensityUnits=kg/m^3  DoExposeReferenceFrame=on  GraphicEmissiveColor=[0.0 0.0 0.0 1.0]  ExportEntireGeometry=off  SerializedFrames=<Frames/>  MarkerShape=Sphere  MarkerSize=10  GraphicType=FromGeometry  InertiaType=CalculateFromGeometry  Mass=1  MassUnits=kg  MomentsOfInertia=[1 1 1]  MomentsOfInertiaUnits=kg*m^2  GraphicOpacity=1.0  ProductsOfInertia=[0 0 0]  ProductsOfInertiaUnits=kg*m^2  GraphicShininess=75  GraphicSpecularColor=[0.5 0.5 0.5 1.0]  GraphicVisPropType=SimpleVisualProperties
  Rigid Transform14 : sm_lib/Frames and Transforms/Rigid Transform  TranslationMethod=StandardAxis  TranslationStandardOffset=40.25  TranslationLengthUnit=mm  TranslationStandardAxis=+Z  TranslationCartesianOffset=[0 0 0]  TranslationROffset=0  TranslationROffsetUnits=m  TranslationZOffset=0  TranslationZOffsetUnits=m  TranslationThetaOffset=0  TranslationThetaOffsetUnits=deg  RotationMethod=None  RotationAngleUnits=deg  RotationStandardAxis=+Z  RotationAngle=0.0  RotationArbitraryAxis=[0 0 1]  FollAlignAxisA=+X  BaseAlignAxisA=+Y  FollAlignAxisB=+Y  BaseAlignAxisB=+Z  RotationSequenceAxes=FollowerAxes  RotationSequence=XYX  RotationSequenceAngles=[0 0 0]  RotationSequenceAnglesUnits=deg  RotationMatrix=[1 0 0; 0 1 0; 0 0 1]
  Conn1 : PMIOPort  Side=Left
  connections:
  Rigid Transform14/RConn1 -- Brick Solid/RConn1
  Rigid Transform14/LConn1 -- Conn1/RConn1

== system base_simulink/Subsystem/base/Manipulator/External Load ==
  Brick Solid : sm_lib/Body Elements/Brick Solid  GraphicAmbientColor=[0.15 0.15 0.15 1.0]  BasedOnType=Mass  BrickDimensions=[50 50 50]  BrickDimensionUnits=mm  CenterOfMass=[0 0 0]  CenterOfMassUnits=m  GraphicDiffuseColor=[0.5 0.5 0.5]  Density=1000  DensityUnits=kg/m^3  DoExposeReferenceFrame=on  GraphicEmissiveColor=[0.0 0.0 0.0 1.0]  ExportEntireGeometry=off  SerializedFrames=<Frames/>  MarkerShape=Sphere  MarkerSize=10  GraphicType=FromGeometry  InertiaType=CalculateFromGeometry  Mass=50  MassUnits=g  MomentsOfInertia=[1 1 1]  MomentsOfInertiaUnits=kg*m^2  GraphicOpacity=1.0  ProductsOfInertia=[0 0 0]  ProductsOfInertiaUnits=kg*m^2  GraphicShininess=75  GraphicSpecularColor=[0.5 0.5 0.5 1.0]  GraphicVisPropType=SimpleVisualProperties
  Rigid Transform14 : sm_lib/Frames and Transforms/Rigid Transform  TranslationMethod=StandardAxis  TranslationStandardOffset=40.25  TranslationLengthUnit=mm  TranslationStandardAxis=+Z  TranslationCartesianOffset=[0 0 0]  TranslationROffset=0  TranslationROffsetUnits=m  TranslationZOffset=0  TranslationZOffsetUnits=m  TranslationThetaOffset=0  TranslationThetaOffsetUnits=deg  RotationMethod=None  RotationAngleUnits=deg  RotationStandardAxis=+Z  RotationAngle=0.0  RotationArbitraryAxis=[0 0 1]  FollAlignAxisA=+X  BaseAlignAxisA=+Y  FollAlignAxisB=+Y  BaseAlignAxisB=+Z  RotationSequenceAxes=FollowerAxes  RotationSequence=XYX  RotationSequenceAngles=[0 0 0]  RotationSequenceAnglesUnits=deg  RotationMatrix=[1 0 0; 0 1 0; 0 0 1]
  Conn1 : PMIOPort  Side=Left
  connections:
  Rigid Transform14/RConn1 -- Brick Solid/RConn1
  Rigid Transform14/LConn1 -- Conn1/RConn1

== matlab function base_simulink/HouseM8/Kalman filter R/Kalman filter ==
  data: theta_k input; X1 output; X1 input; X2 input; P11 input; P12 input; P21 input; P22 input; X2 output; PP11 output; PP12 output; PP21 output; PP22 output; dP output
function [X1,X2,PP11,PP12,PP21,PP22,dP] = KalmanFilterFNC(theta_k,X1,X2,P11,P12,P21,P22)
%syms delta_t theta_k omega_k V_k Q x_k1 xp_hat_k x_hat_k P_hat_k yp_k R x11 x21 p11 p12 p21 p22 dt
dt = 0.0001;
omega_k = 0;
delta_t = dt;
A = [1 delta_t;0 1];
G = [delta_t*delta_t/2;delta_t];
C = [1 0];
Q = 6.800;
R = 0.01;
x_k = [theta_k;0]
%x_k = A*x_k1;
y_k = C*x_k;
x11 = X1;
x21 = X2;
x_hat_k = [x11;x21]
p11 = P11;
p12 = P12;
p21 = P21;
p22 = P22;
P_hat_k = [p11 p12;p21 p22];

%pred -------------------------------------

xp_hat_k = A*x_hat_k;
Pp_hat_k = A*P_hat_k*transpose(A) + G*Q*transpose(G);

%upadate

yp_k = C*xp_hat_k;
y_re_k = y_k - yp_k;
S_k = C*Pp_hat_k*transpose(C) + R;
K_k = Pp_hat_k*transpose(C)/(S_k);
x_hat_k1 = xp_hat_k+K_k*y_re_k;
P_hat_k1 = ([1 0;0 1]-(K_k*C))*Pp_hat_k;

%X1 = x_hat_k1(1);
%X2 = x_hat_k1(2);
%PP11 = P_hat_k1(1,1);
%PP12 = P_hat_k1(1,2);
%PP21 = P_hat_k1(2,1);
%PP22 =P_hat_k1(2,2);
X1 = X1 + X2*dt - ((X1 - theta_k + X2*dt)*(P11 + P21*dt + (Q*dt^4)/4 + dt*(P12 + P22*dt)))/(P11 + R + P21*dt + (Q*(dt^4))/4 + dt*(P12 + P22*dt));
X2 = X2 - (((Q*(dt^3))/2 + P22*dt + P21)*(X1 - theta_k + X2*dt))/(P11 + R + P21*dt + (Q*(dt^4))/4 + dt*(P12 + P22*dt));
PP11 = -((P11 + P21*dt + (Q*(dt^4))/4 + dt*(P12 + P22*dt))/(P11 + R + P21*dt + (Q*(dt^4))/4 + dt*(P12 + P22*dt)) - 1)*(P11 + P21*dt + (Q*(dt^4))/4 + dt*(P12 + P22*dt));
PP12 = -((P11 + P21*dt + (Q*(dt^4))/4 + dt*(P12 + P22*dt))/(P11 + R + P21*dt + (Q*(dt^4))/4 + dt*(P12 + P22*dt)) - 1)*((Q*(dt^3))/2 + P22*dt + P12);
PP21 = P21 + P22*dt + (Q*(dt^3))/2 - (((Q*(dt^3))/2 + P22*dt + P21)*(P11 + P21*dt + (Q*(dt^4))/4 + dt*(P12 + P22*dt)))/(P11 + R + P21*dt + (Q*(dt^4))/4 + dt*(P12 + P22*dt));
PP22 = P22 + Q*(dt^2) - (((Q*(dt^3))/2 + P22*dt + P12)*((Q*(dt^3))/2 + P22*dt + P21))/(P11 + R + P21*dt + (Q*(dt^4))/4 + dt*(P12 + P22*dt));
dP = det([PP11 PP12;PP21 PP22])

== matlab function base_simulink/HouseM8/MATLAB Function ==
  data: wL input; v output; wR input; R input; L input; w output
function [v,w] = FK(wL,wR,R,L)
v = (R/2)*(wL+wR);
w = (R/L)*(wR-wL);

== matlab function base_simulink/Traj ==
  data: q0 input; qd output; qf input; v0 input; qv output; qa output; T output; t input
function [qd,qv,qa,T] = GenTraj(q0,qf,v0,t) % vf ,ai , af =0 
    t0 = 0;
%     vmax = pi/2;
% 
%     dq = qf - q0;
%     tf = abs(dq/((vmax-v0)/1.9));

%     t = linspace(t0,tf,1000*(tf - t0));
    tf=0.1;
    T = tf;
    
    ds = q0 - qf;
    tfv0 = tf*v0;

    co0 = q0;
    co1 = v0;
    co2 = 0;
    co3 =  - (2*(5*ds + 3*(tfv0)))/tf^3;
    co4 = (15*ds + 8*tfv0)/tf^4;
    co5 =  - (3*(2*ds + tfv0))/tf^5;

    qd = co0 + (co1.*t) + (co3.*t.^3) + (co4.*t.^4) + (co5.*t.^5);
    qv = co1 + (3*co3.*t.^2) + (4*co4.*t.^3) + (5*co5.*t.^4);
    qa = (6*co3.*t) + (12*co4.*t.^2) + (20*co5.*t.^3);
end

== matlab function base_simulink/Traj1 ==
  data: q0 input; qd output; qf input; v0 input; qv output; qa output; T output; t input
function [qd,qv,qa,T] = GenTraj(q0,qf,v0,t) % vf ,ai , af =0 
    t0 = 0;
%     vmax = pi/2;
% 
%     dq = qf - q0;
%     tf = abs(dq/((vmax-v0)/1.9));

%     t = linspace(t0,tf,1000*(tf - t0));
    tf=10;
    T = tf;
    
    ds = q0 - qf;
    tfv0 = tf*v0;

    co0 = q0;
    co1 = v0;
    co2 = 0;
    co3 =  - (2*(5*ds + 3*(tfv0)))/tf^3;
    co4 = (15*ds + 8*tfv0)/tf^4;
    co5 =  - (3*(2*ds + tfv0))/tf^5;

    qd = co0 + (co1.*t) + (co3.*t.^3) + (co4.*t.^4) + (co5.*t.^5);
    qv = co1 + (3*co3.*t.^2) + (4*co4.*t.^3) + (5*co5.*t.^4);
    qa = (6*co3.*t) + (12*co4.*t.^2) + (20*co5.*t.^3);
end

== matlab function base_simulink/Subsystem/Kalman filter L/Kalman filter ==
  data: theta_k input; X1 output; X1 input; X2 input; P11 input; P12 input; P21 input; P22 input; X2 output; PP11 output; PP12 output; PP21 output; PP22 output; dP output
function [X1,X2,PP11,PP12,PP21,PP22,dP] = KalmanFilterFNC(theta_k,X1,X2,P11,P12,P21,P22)
%syms delta_t theta_k omega_k V_k Q x_k1 xp_hat_k x_hat_k P_hat_k yp_k R x11 x21 p11 p12 p21 p22 dt
dt = 0.0001;
omega_k = 0;
delta_t = dt;
A = [1 delta_t;0 1];
G = [delta_t*delta_t/2;delta_t];
C = [1 0];
Q = 6.800;
R = 0.01;
x_k = [theta_k;0]
%x_k = A*x_k1;
y_k = C*x_k;
x11 = X1;
x21 = X2;
x_hat_k = [x11;x21]
p11 = P11;
p12 = P12;
p21 = P21;
p22 = P22;
P_hat_k = [p11 p12;p21 p22];

%pred -------------------------------------

xp_hat_k = A*x_hat_k;
Pp_hat_k = A*P_hat_k*transpose(A) + G*Q*transpose(G);

%upadate

yp_k = C*xp_hat_k;
y_re_k = y_k - yp_k;
S_k = C*Pp_hat_k*transpose(C) + R;
K_k = Pp_hat_k*transpose(C)/(S_k);
x_hat_k1 = xp_hat_k+K_k*y_re_k;
P_hat_k1 = ([1 0;0 1]-(K_k*C))*Pp_hat_k;

%X1 = x_hat_k1(1);
%X2 = x_hat_k1(2);
%PP11 = P_hat_k1(1,1);
%PP12 = P_hat_k1(1,2);
%PP21 = P_hat_k1(2,1);
%PP22 =P_hat_k1(2,2);
X1 = X1 + X2*dt - ((X1 - theta_k + X2*dt)*(P11 + P21*dt + (Q*dt^4)/4 + dt*(P12 + P22*dt)))/(P11 + R + P21*dt + (Q*(dt^4))/4 + dt*(P12 + P22*dt));
X2 = X2 - (((Q*(dt^3))/2 + P22*dt + P21)*(X1 - theta_k + X2*dt))/(P11 + R + P21*dt + (Q*(dt^4))/4 + dt*(P12 + P22*dt));
PP11 = -((P11 + P21*dt + (Q*(dt^4))/4 + dt*(P12 + P22*dt))/(P11 + R + P21*dt + (Q*(dt^4))/4 + dt*(P12 + P22*dt)) - 1)*(P11 + P21*dt + (Q*(dt^4))/4 + dt*(P12 + P22*dt));
PP12 = -((P11 + P21*dt + (Q*(dt^4))/4 + dt*(P12 + P22*dt))/(P11 + R + P21*dt + (Q*(dt^4))/4 + dt*(P12 + P22*dt)) - 1)*((Q*(dt^3))/2 + P22*dt + P12);
PP21 = P21 + P22*dt + (Q*(dt^3))/2 - (((Q*(dt^3))/2 + P22*dt + P21)*(P11 + P21*dt + (Q*(dt^4))/4 + dt*(P12 + P22*dt)))/(P11 + R + P21*dt + (Q*(dt^4))/4 + dt*(P12 + P22*dt));
PP22 = P22 + Q*(dt^2) - (((Q*(dt^3))/2 + P22*dt + P12)*((Q*(dt^3))/2 + P22*dt + P21))/(P11 + R + P21*dt + (Q*(dt^4))/4 + dt*(P12 + P22*dt));
dP = det([PP11 PP12;PP21 PP22])

== matlab function base_simulink/Subsystem/IK ==
  data: v input; wL output; w input; R input; L input; wR output
function [wL,wR] = IK(v,w,R,L)
wL = (1/R)*(v-(w*L)/2);
wR = (1/R)*(v+(w*L)/2);

== matlab function base_simulink/Subsystem/Kalman filter R/Kalman filter ==
  data: theta_k input; X1 output; X1 input; X2 input; P11 input; P12 input; P21 input; P22 input; X2 output; PP11 output; PP12 output; PP21 output; PP22 output; dP output
function [X1,X2,PP11,PP12,PP21,PP22,dP] = KalmanFilterFNC(theta_k,X1,X2,P11,P12,P21,P22)
%syms delta_t theta_k omega_k V_k Q x_k1 xp_hat_k x_hat_k P_hat_k yp_k R x11 x21 p11 p12 p21 p22 dt
dt = 0.0001;
omega_k = 0;
delta_t = dt;
A = [1 delta_t;0 1];
G = [delta_t*delta_t/2;delta_t];
C = [1 0];
Q = 6.800;
R = 0.01;
x_k = [theta_k;0]
%x_k = A*x_k1;
y_k = C*x_k;
x11 = X1;
x21 = X2;
x_hat_k = [x11;x21]
p11 = P11;
p12 = P12;
p21 = P21;
p22 = P22;
P_hat_k = [p11 p12;p21 p22];

%pred -------------------------------------

xp_hat_k = A*x_hat_k;
Pp_hat_k = A*P_hat_k*transpose(A) + G*Q*transpose(G);

%upadate

yp_k = C*xp_hat_k;
y_re_k = y_k - yp_k;
S_k = C*Pp_hat_k*transpose(C) + R;
K_k = Pp_hat_k*transpose(C)/(S_k);
x_hat_k1 = xp_hat_k+K_k*y_re_k;
P_hat_k1 = ([1 0;0 1]-(K_k*C))*Pp_hat_k;

%X1 = x_hat_k1(1);
%X2 = x_hat_k1(2);
%PP11 = P_hat_k1(1,1);
%PP12 = P_hat_k1(1,2);
%PP21 = P_hat_k1(2,1);
%PP22 =P_hat_k1(2,2);
X1 = X1 + X2*dt - ((X1 - theta_k + X2*dt)*(P11 + P21*dt + (Q*dt^4)/4 + dt*(P12 + P22*dt)))/(P11 + R + P21*dt + (Q*(dt^4))/4 + dt*(P12 + P22*dt));
X2 = X2 - (((Q*(dt^3))/2 + P22*dt + P21)*(X1 - theta_k + X2*dt))/(P11 + R + P21*dt + (Q*(dt^4))/4 + dt*(P12 + P22*dt));
PP11 = -((P11 + P21*dt + (Q*(dt^4))/4 + dt*(P12 + P22*dt))/(P11 + R + P21*dt + (Q*(dt^4))/4 + dt*(P12 + P22*dt)) - 1)*(P11 + P21*dt + (Q*(dt^4))/4 + dt*(P12 + P22*dt));
PP12 = -((P11 + P21*dt + (Q*(dt^4))/4 + dt*(P12 + P22*dt))/(P11 + R + P21*dt + (Q*(dt^4))/4 + dt*(P12 + P22*dt)) - 1)*((Q*(dt^3))/2 + P22*dt + P12);
PP21 = P21 + P22*dt + (Q*(dt^3))/2 - (((Q*(dt^3))/2 + P22*dt + P21)*(P11 + P21*dt + (Q*(dt^4))/4 + dt*(P12 + P22*dt)))/(P11 + R + P21*dt + (Q*(dt^4))/4 + dt*(P12 + P22*dt));
PP22 = P22 + Q*(dt^2) - (((Q*(dt^3))/2 + P22*dt + P12)*((Q*(dt^3))/2 + P22*dt + P21))/(P11 + R + P21*dt + (Q*(dt^4))/4 + dt*(P12 + P22*dt));
dP = det([PP11 PP12;PP21 PP22])

== matlab function base_simulink/Subsystem/MATLAB Function ==
  data: wL input; v output; wR input; R input; L input; w output
function [v,w] = FK(wL,wR,R,L)
v = (R/2)*(wL+wR);
w = (R/L)*(wR-wL);

== matlab function base_simulink/HouseM8/IK ==
  data: v input; wL output; w input; R input; L input; wR output
function [wL,wR] = IK(v,w,R,L)
wL = (1/R)*(v-(w*L)/2);
wR = (1/R)*(v+(w*L)/2);

== matlab function base_simulink/HouseM8/Kalman filter L/Kalman filter ==
  data: theta_k input; X1 output; X1 input; X2 input; P11 input; P12 input; P21 input; P22 input; X2 output; PP11 output; PP12 output; PP21 output; PP22 output; dP output
function [X1,X2,PP11,PP12,PP21,PP22,dP] = KalmanFilterFNC(theta_k,X1,X2,P11,P12,P21,P22)
%syms delta_t theta_k omega_k V_k Q x_k1 xp_hat_k x_hat_k P_hat_k yp_k R x11 x21 p11 p12 p21 p22 dt
dt = 0.0001;
omega_k = 0;
delta_t = dt;
A = [1 delta_t;0 1];
G = [delta_t*delta_t/2;delta_t];
C = [1 0];
Q = 6.800;
R = 0.01;
x_k = [theta_k;0]
%x_k = A*x_k1;
y_k = C*x_k;
x11 = X1;
x21 = X2;
x_hat_k = [x11;x21]
p11 = P11;
p12 = P12;
p21 = P21;
p22 = P22;
P_hat_k = [p11 p12;p21 p22];

%pred -------------------------------------

xp_hat_k = A*x_hat_k;
Pp_hat_k = A*P_hat_k*transpose(A) + G*Q*transpose(G);

%upadate

yp_k = C*xp_hat_k;
y_re_k = y_k - yp_k;
S_k = C*Pp_hat_k*transpose(C) + R;
K_k = Pp_hat_k*transpose(C)/(S_k);
x_hat_k1 = xp_hat_k+K_k*y_re_k;
P_hat_k1 = ([1 0;0 1]-(K_k*C))*Pp_hat_k;

%X1 = x_hat_k1(1);
%X2 = x_hat_k1(2);
%PP11 = P_hat_k1(1,1);
%PP12 = P_hat_k1(1,2);
%PP21 = P_hat_k1(2,1);
%PP22 =P_hat_k1(2,2);
X1 = X1 + X2*dt - ((X1 - theta_k + X2*dt)*(P11 + P21*dt + (Q*dt^4)/4 + dt*(P12 + P22*dt)))/(P11 + R + P21*dt + (Q*(dt^4))/4 + dt*(P12 + P22*dt));
X2 = X2 - (((Q*(dt^3))/2 + P22*dt + P21)*(X1 - theta_k + X2*dt))/(P11 + R + P21*dt + (Q*(dt^4))/4 + dt*(P12 + P22*dt));
PP11 = -((P11 + P21*dt + (Q*(dt^4))/4 + dt*(P12 + P22*dt))/(P11 + R + P21*dt + (Q*(dt^4))/4 + dt*(P12 + P22*dt)) - 1)*(P11 + P21*dt + (Q*(dt^4))/4 + dt*(P12 + P22*dt));
PP12 = -((P11 + P21*dt + (Q*(dt^4))/4 + dt*(P12 + P22*dt))/(P11 + R + P21*dt + (Q*(dt^4))/4 + dt*(P12 + P22*dt)) - 1)*((Q*(dt^3))/2 + P22*dt + P12);
PP21 = P21 + P22*dt + (Q*(dt^3))/2 - (((Q*(dt^3))/2 + P22*dt + P21)*(P11 + P21*dt + (Q*(dt^4))/4 + dt*(P12 + P22*dt)))/(P11 + R + P21*dt + (Q*(dt^4))/4 + dt*(P12 + P22*dt));
PP22 = P22 + Q*(dt^2) - (((Q*(dt^3))/2 + P22*dt + P12)*((Q*(dt^3))/2 + P22*dt + P21))/(P11 + R + P21*dt + (Q*(dt^4))/4 + dt*(P12 + P22*dt));
dP = det([PP11 PP12;PP21 PP22])
